simulink model "circuitss"  (R2015a)
settings: Solver=ode45  StartTime=0.0  StopTime=10.0  RelTol=1e-3
values from neighbouring files (symbols this model uses):
  Cap = x * 1000e-6    (= 0.01)    [circex.m]
  L = y * 100e-3    (= 1)    [circex.m]
  R = z    (= 10)    [circex.m]
settings Model: Creator=eechris  LastModifiedBy=eechris
settings DataIOCC: SignalLoggingSaveFormat=ModelDataLogs
settings OptimizationCC: ExpressionDepthLimit=2147483647
settings DebuggingCC: UnderspecifiedInitializationDetection=Classic  MergeDetectMultiDrivingBlocksExec=none  SolverPrmCheckMsg=warning  FcnCallInpInsideContextMsg=UseLocalSettings  StateNameClashWarn=warning  StrictBusMsg=Warning
settings GRTTargetCC: CombineOutputUpdateFcns=off  GRTInterface=on

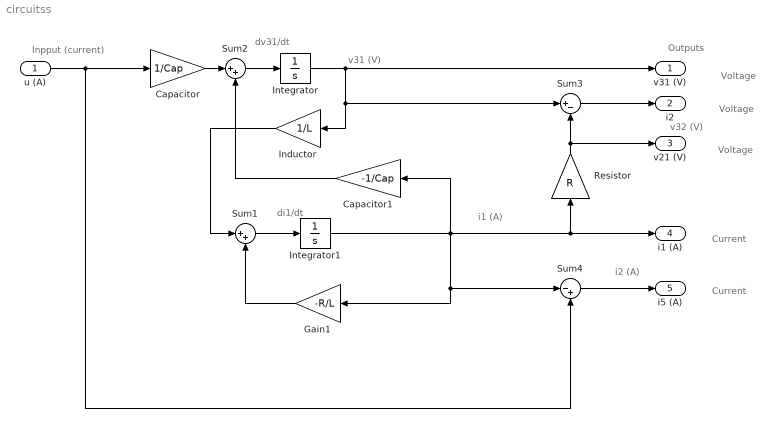
== system circuitss ==
  note: dv31/dt
  note: v31 (V)
  note: v32 (V)
  note: di1/dt
  note: i1 (A)
  note: i2 (A)
  note: Inpput (current)
  note: Outputs
  note: Voltage
  note: Voltage
  note: Voltage
  note: Current
  note: Current
  u (A) : Inport
  Capacitor : Gain  Gain=1/Cap
  Capacitor1 : Gain  Gain=-1/Cap
  Gain1 : Gain  Gain=-R/L
  Inductor : Gain  Gain=1/L
  Integrator : Integrator
  Integrator1 : Integrator
  Resistor : Gain  Gain=R
  Sum1 : Sum  Inputs=|++
  Sum2 : Sum  Inputs=|++
  Sum3 : Sum  Inputs=|+-
  Sum4 : Sum  Inputs=|-+
  v31 (V) : Outport
  i2 : Outport  Port=2
  v21 (V) : Outport  Port=3
  i1 (A) : Outport  Port=4
  i5 (A) : Outport  Port=5
  wires:
  Integrator/1 -> Inductor/1, Sum3/1, v31 (V)/1
  Capacitor/1 -> Sum2/1
  Sum2/1 -> Integrator/1
  Inductor/1 -> Sum1/1
  Sum1/1 -> Integrator1/1
  Gain1/1 -> Sum1/2
  Capacitor1/1 -> Sum2/2
  u (A)/1 -> Capacitor/1, Sum4/2
  Resistor/1 -> Sum3/2, v21 (V)/1
  Sum3/1 -> i2/1
  Integrator1/1 -> Capacitor1/1, i1 (A)/1, Resistor/1, Gain1/1, Sum4/1
  Sum4/1 -> i5 (A)/1
